simulink model "Design_5new_4weeks_01_06_MQTT"  (R2026a)
settings: Solver=FixedStepAuto  StopTime=2419200  FixedStep=300
undefined symbols (not defined in the file): m, n
libraries: mqttlib x7
(part 2 of 2)

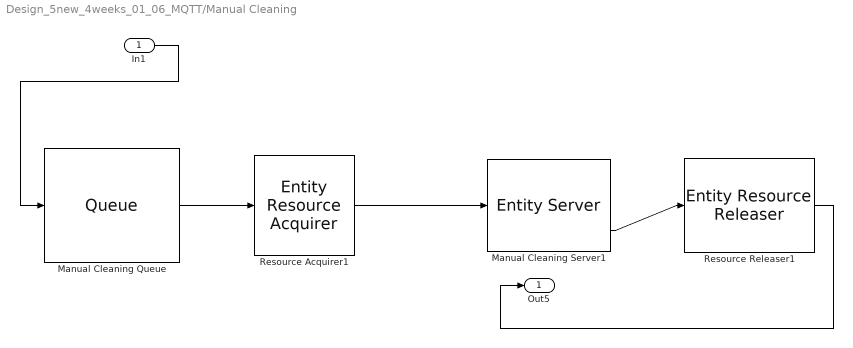
== system Design_5new_4weeks_01_06_MQTT/Manual Cleaning ==
  In1 : Inport
  Manual Cleaning Queue : Queue  InputPortMessageModes=m  OutputPortMessageModes=m
  Manual Cleaning Server1 : EntityServer  InputPortMessageModes=m  OutputPortMessageModes=n,m  Capacity=1  ServiceTimeValue=30*60  EntryAction=|  NumberEntitiesDeparted=on
      | %#codegen
      | 
      | % =========================================================
      | % MANUAL CLEANING PROCESS
      | % Supervisor Excel Values
      | % Simulink-safe version
      | % =========================================================
      | 
      | % Manual Cleaning completed
      | entity.prev_proc = 4;
      | 
      | % =========================================================
      | % FIX MANUAL BATCH ID
      | % =========================================================
      | % In the model, ManualBatchID sometimes becomes 0 here.
      | % If it is 0, use BatchID as the correct ManualBatchID.
      | % =========================================================
      | 
      | if entity.ManualBatchID == 0
      |     entity.ManualBatchID = entity.BatchID;
      | end
      | 
      | % =========================================================
      | % SUPERVISOR VALUES
      | % =========================================================
      | 
      | entity.operator_time_min = 30;              % min/batch
      | entity.capacity_L        = entity.part_volume;
      | entity.process_time_min  = 30;              % min
      | entity.power             = 0;               % kW
      | 
      | % =========================================================
      | % ENERGY CALCULATION
      | % =========================================================
      | 
      | entity.energy = 0;                          % kWh
      | 
      | % =========================================================
      | % ACCUMULATE TOTALS
      | % =========================================================
      | 
      | entity.total_energy = ...
      |     entity.total_energy + entity.energy;
      | 
      | entity.total_operator_min = ...
      |     entity.total_operator_min + entity.operator_time_min;
      | 
      | % =========================================================
      | % DEBUG PRINT
      | % =========================================================
      | 
      | fprintf(['[MANUAL CLEANING CHECK] ' ...
      |     'SourceID=%g | BuildID=%g | BatchID=%g | ' ...
      |     'ManualBatchID=%g | PartID=%g | ' ...
      |     'PrevProc=%g | Volume=%.2f | Capacity=%.2f | ' ...
      |     'ProcessTime=%.2f min | Operator=%.2f min | ' ...
      |     'Power=%.2f kW | Energy=%.3f kWh | ' ...
      |     'TotalEnergy=%.3f kWh | TotalOperator=%.3f min\n'], ...
      |     entity.SourceID, ...
      |     entity.BuildID, ...
      |     entity.BatchID, ...
      |     entity.ManualBatchID, ...
      |     entity.PartID, ...
      |     entity.prev_proc, ...
      |     entity.part_volume, ...
      |     entity.capacity_L, ...
      |     entity.process_time_min, ...
      |     entity.operator_time_min, ...
      |     entity.power, ...
      |     entity.energy, ...
      |     entity.total_energy, ...
      |     entity.total_operator_min);
      | 
      | % =========================================================
      | % MQTT PAYLOAD - MANUAL CLEANING
      | % FIWARE JSON object format
      | % =========================================================
      | 
      | payload = sprintf( ...
      |     '{"BuildID":%.0f,"BatchID":%.0f,"ManualBatchID":%.0f,"PartID":%.0f,"Volume":%.2f,"ProcessTime":%.2f,"Energy":%.3f}', ...
      |     entity.BuildID, ...
      |     entity.BatchID, ...
      |     entity.ManualBatchID, ...
      |     entity.PartID, ...
      |     entity.part_volume, ...
      |     entity.process_time_min, ...
      |     entity.energy);
      | 
      | payload = char(payload);
      | 
      | disp("[MANUAL CLEANING MQTT PAYLOAD]")
      | disp(payload)
      | 
      | % =========================================================
      | % CALL SIMULINK FUNCTION FOR MQTT PUBLISH
      | % This sends payload to MQTT Publish block
      | % =========================================================
      | 
      | publishManualCleaning( ...
      |     entity.BuildID, ...
      |     entity.BatchID, ...
      |     entity.ManualBatchID, ...
      |     entity.PartID, ...
      |     entity.part_volume, ...
      |     entity.process_time_min, ...
      |     entity.energy);
      settings: OutputPortMap=o0,o9
  Resource Acquirer1 : EntityResourceAcquirer  InputPortMessageModes=m  OutputPortMessageModes=m  ResourceName=operator_pool_1
      settings: OutputPortMap=o3
  Resource Releaser1 : EntityResourceReleaser  InputPortMessageModes=m  OutputPortMessageModes=m
  Out5 : Outport
  wires:
  Manual Cleaning Server1/2 -> Resource Releaser1/1
  In1/1 -> Manual Cleaning Queue/1
  Resource Acquirer1/1 -> Manual Cleaning Server1/1
  Manual Cleaning Queue/1 -> Resource Acquirer1/1
  Resource Releaser1/1 -> Out5/1

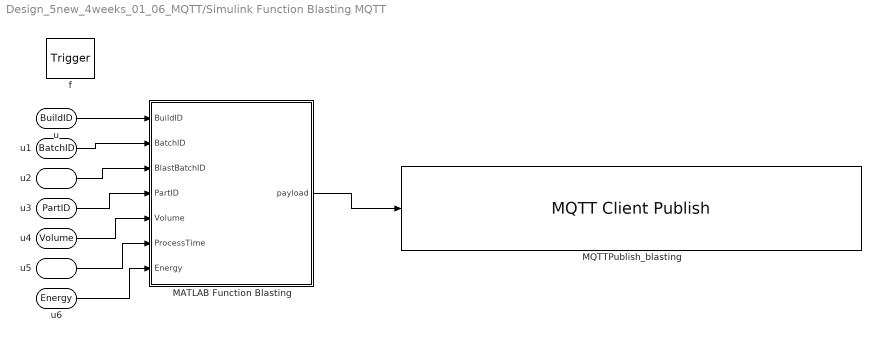
== system Design_5new_4weeks_01_06_MQTT/Simulink Function Blasting MQTT ==
  f : TriggerPort  TriggerType=function-call  IsSimulinkFunction=on  FunctionName=publishBlasting  VariantControl=(inherit)
  MATLAB Function Blasting : MATLAB Function  TreatAsAtomicUnit=on
  MQTTPublish_blasting : mqttlib/MQTT Client Publish  RetainClient=Fiware 1  ClientList=Fiware 1  TopicsTable={ '1', 'json/SLSProcess/BlastingMachine:001/attrs', '0', 'off' }  PublishOnDataChange=off  SampleTime=-1  TopicNames=json/SLSProcess/BlastingMachine:001/attrs  NumTopics=1  IsLib=0  BlkName=MQTT Client Publish
  u : ArgIn  DisableCoverage=on  ArgumentName=BuildID
  u1 : ArgIn  DisableCoverage=on  Port=2  ArgumentName=BatchID
  u2 : ArgIn  DisableCoverage=on  Port=3  ArgumentName=BlastBatchID
  u3 : ArgIn  DisableCoverage=on  Port=4  ArgumentName=PartID
  u4 : ArgIn  DisableCoverage=on  Port=5  ArgumentName=Volume
  u5 : ArgIn  DisableCoverage=on  Port=6  ArgumentName=ProcessTime
  u6 : ArgIn  DisableCoverage=on  Port=7  ArgumentName=Energy
  wires:
  u/1 -> MATLAB Function Blasting/1(BuildID)
  u1/1 -> MATLAB Function Blasting/2(BatchID)
  u2/1 -> MATLAB Function Blasting/3(BlastBatchID)
  u3/1 -> MATLAB Function Blasting/4(PartID)
  u4/1 -> MATLAB Function Blasting/5(Volume)
  u5/1 -> MATLAB Function Blasting/6(ProcessTime)
  u6/1 -> MATLAB Function Blasting/7(Energy)
  MATLAB Function Blasting/1(payload) -> MQTTPublish_blasting/1

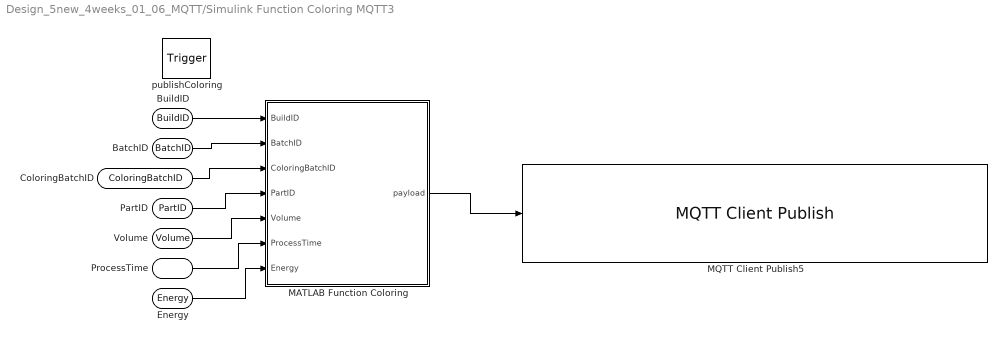
== system Design_5new_4weeks_01_06_MQTT/Simulink Function Coloring MQTT3 ==
  publishColoring : TriggerPort  TriggerType=function-call  IsSimulinkFunction=on  FunctionName=publishColoring  VariantControl=(inherit)
  MATLAB Function Coloring : MATLAB Function  TreatAsAtomicUnit=on
  MQTT Client Publish5 : mqttlib/MQTT Client Publish  RetainClient=Fiware 1  ClientList=Fiware 1  TopicsTable={ '1', 'json/SLSProcess/ColoringMachine:001/attrs', '0', 'off' }  PublishOnDataChange=off  SampleTime=-1  TopicNames=json/SLSProcess/ColoringMachine:001/attrs  NumTopics=1  IsLib=0  BlkName=MQTT Client Publish
  BuildID : ArgIn  DisableCoverage=on  ArgumentName=BuildID
  BatchID : ArgIn  DisableCoverage=on  Port=2  ArgumentName=BatchID
  ColoringBatchID : ArgIn  DisableCoverage=on  Port=3  ArgumentName=ColoringBatchID
  PartID : ArgIn  DisableCoverage=on  Port=4  ArgumentName=PartID
  Volume : ArgIn  DisableCoverage=on  Port=5  ArgumentName=Volume
  ProcessTime : ArgIn  DisableCoverage=on  Port=6  ArgumentName=ProcessTime
  Energy : ArgIn  DisableCoverage=on  Port=7  ArgumentName=Energy
  wires:
  BuildID/1 -> MATLAB Function Coloring/1(BuildID)
  BatchID/1 -> MATLAB Function Coloring/2(BatchID)
  ColoringBatchID/1 -> MATLAB Function Coloring/3(ColoringBatchID)
  PartID/1 -> MATLAB Function Coloring/4(PartID)
  Volume/1 -> MATLAB Function Coloring/5(Volume)
  ProcessTime/1 -> MATLAB Function Coloring/6(ProcessTime)
  Energy/1 -> MATLAB Function Coloring/7(Energy)
  MATLAB Function Coloring/1(payload) -> MQTT Client Publish5/1

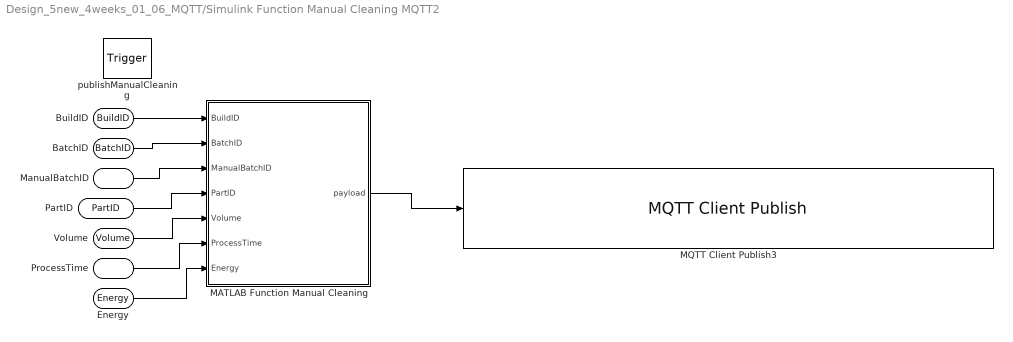
== system Design_5new_4weeks_01_06_MQTT/Simulink Function Manual Cleaning MQTT2 ==
  publishManualCleaning : TriggerPort  TriggerType=function-call  IsSimulinkFunction=on  FunctionName=publishManualCleaning  VariantControl=(inherit)
  MATLAB Function Manual Cleaning : MATLAB Function  TreatAsAtomicUnit=on
  MQTT Client Publish3 : mqttlib/MQTT Client Publish  RetainClient=Fiware 1  ClientList=Fiware 1  TopicsTable={ '1', 'json/SLSProcess/ManualCleaningMachine:001/attrs', '0', 'off' }  PublishOnDataChange=off  SampleTime=-1  TopicNames=json/SLSProcess/ManualCleaningMachine:001/attrs  NumTopics=1  IsLib=0  BlkName=MQTT Client Publish
  BuildID : ArgIn  DisableCoverage=on  ArgumentName=BuildID
  BatchID : ArgIn  DisableCoverage=on  Port=2  ArgumentName=BatchID
  ManualBatchID : ArgIn  DisableCoverage=on  Port=3  ArgumentName=ManualBatchID
  PartID : ArgIn  DisableCoverage=on  Port=4  ArgumentName=PartID
  Volume : ArgIn  DisableCoverage=on  Port=5  ArgumentName=Volume
  ProcessTime : ArgIn  DisableCoverage=on  Port=6  ArgumentName=ProcessTime
  Energy : ArgIn  DisableCoverage=on  Port=7  ArgumentName=Energy
  wires:
  BuildID/1 -> MATLAB Function Manual Cleaning/1(BuildID)
  BatchID/1 -> MATLAB Function Manual Cleaning/2(BatchID)
  ManualBatchID/1 -> MATLAB Function Manual Cleaning/3(ManualBatchID)
  PartID/1 -> MATLAB Function Manual Cleaning/4(PartID)
  Volume/1 -> MATLAB Function Manual Cleaning/5(Volume)
  ProcessTime/1 -> MATLAB Function Manual Cleaning/6(ProcessTime)
  Energy/1 -> MATLAB Function Manual Cleaning/7(Energy)
  MATLAB Function Manual Cleaning/1(payload) -> MQTT Client Publish3/1

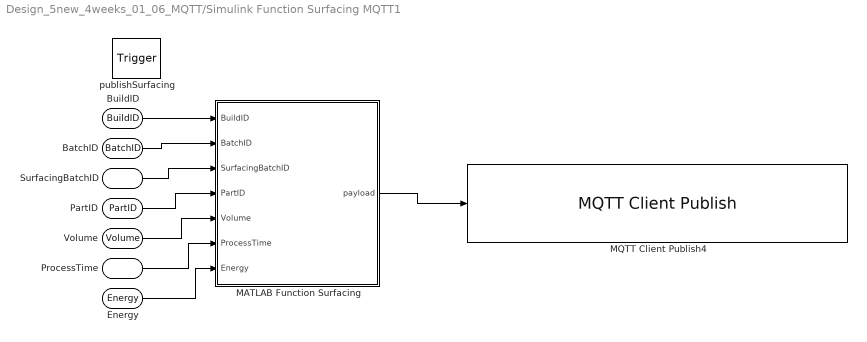
== system Design_5new_4weeks_01_06_MQTT/Simulink Function Surfacing MQTT1 ==
  publishSurfacing : TriggerPort  TriggerType=function-call  IsSimulinkFunction=on  FunctionName=publishSurfacing  VariantControl=(inherit)
  MATLAB Function Surfacing : MATLAB Function  TreatAsAtomicUnit=on
  MQTT Client Publish4 : mqttlib/MQTT Client Publish  RetainClient=Fiware 1  ClientList=Fiware 1  TopicsTable={ '1', 'json/SLSProcess/SurfacingMachine:001/attrs', '0', 'off' }  PublishOnDataChange=off  SampleTime=-1  TopicNames=json/SLSProcess/SurfacingMachine:001/attrs  NumTopics=1  IsLib=0  BlkName=MQTT Client Publish
  BuildID : ArgIn  DisableCoverage=on  ArgumentName=BuildID
  BatchID : ArgIn  DisableCoverage=on  Port=2  ArgumentName=BatchID
  SurfacingBatchID : ArgIn  DisableCoverage=on  Port=3  ArgumentName=SurfacingBatchID
  PartID : ArgIn  DisableCoverage=on  Port=4  ArgumentName=PartID
  Volume : ArgIn  DisableCoverage=on  Port=5  ArgumentName=Volume
  ProcessTime : ArgIn  DisableCoverage=on  Port=6  ArgumentName=ProcessTime
  Energy : ArgIn  DisableCoverage=on  Port=7  ArgumentName=Energy
  wires:
  BuildID/1 -> MATLAB Function Surfacing/1(BuildID)
  BatchID/1 -> MATLAB Function Surfacing/2(BatchID)
  SurfacingBatchID/1 -> MATLAB Function Surfacing/3(SurfacingBatchID)
  PartID/1 -> MATLAB Function Surfacing/4(PartID)
  Volume/1 -> MATLAB Function Surfacing/5(Volume)
  ProcessTime/1 -> MATLAB Function Surfacing/6(ProcessTime)
  Energy/1 -> MATLAB Function Surfacing/7(Energy)
  MATLAB Function Surfacing/1(payload) -> MQTT Client Publish4/1

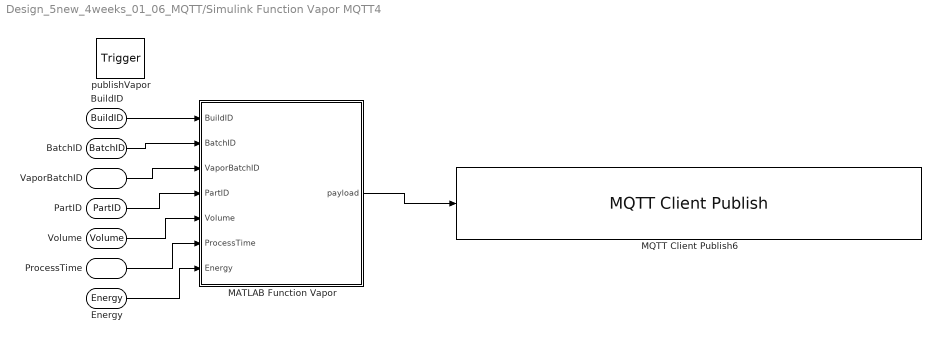
== system Design_5new_4weeks_01_06_MQTT/Simulink Function Vapor MQTT4 ==
  publishVapor : TriggerPort  TriggerType=function-call  IsSimulinkFunction=on  FunctionName=publishVapor  VariantControl=(inherit)
  MATLAB Function Vapor : MATLAB Function  TreatAsAtomicUnit=on
  MQTT Client Publish6 : mqttlib/MQTT Client Publish  RetainClient=Fiware 1  ClientList=Fiware 1  TopicsTable={ '1', 'json/SLSProcess/VaporSmoothingMachine:001/attrs', '0', 'off' }  PublishOnDataChange=off  SampleTime=-1  TopicNames=json/SLSProcess/VaporSmoothingMachine:001/attrs  NumTopics=1  IsLib=0  BlkName=MQTT Client Publish
  BuildID : ArgIn  DisableCoverage=on  ArgumentName=BuildID
  BatchID : ArgIn  DisableCoverage=on  Port=2  ArgumentName=BatchID
  VaporBatchID : ArgIn  DisableCoverage=on  Port=3  ArgumentName=VaporBatchID
  PartID : ArgIn  DisableCoverage=on  Port=4  ArgumentName=PartID
  Volume : ArgIn  DisableCoverage=on  Port=5  ArgumentName=Volume
  ProcessTime : ArgIn  DisableCoverage=on  Port=6  ArgumentName=ProcessTime
  Energy : ArgIn  DisableCoverage=on  Port=7  ArgumentName=Energy
  wires:
  BuildID/1 -> MATLAB Function Vapor/1(BuildID)
  BatchID/1 -> MATLAB Function Vapor/2(BatchID)
  VaporBatchID/1 -> MATLAB Function Vapor/3(VaporBatchID)
  PartID/1 -> MATLAB Function Vapor/4(PartID)
  Volume/1 -> MATLAB Function Vapor/5(Volume)
  ProcessTime/1 -> MATLAB Function Vapor/6(ProcessTime)
  Energy/1 -> MATLAB Function Vapor/7(Energy)
  MATLAB Function Vapor/1(payload) -> MQTT Client Publish6/1

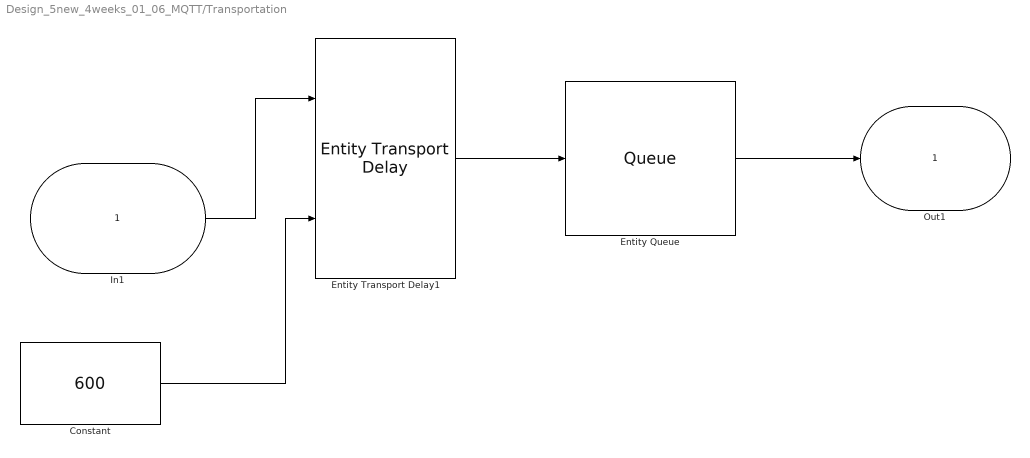
== system Design_5new_4weeks_01_06_MQTT/Transportation ==
  In1 : Inport
  Constant : Constant  Value=600
  Entity Transport Delay1 : EntityTransportDelay  InputPortMessageModes=m,n  OutputPortMessageModes=m
  Entity Queue : Queue  InputPortMessageModes=m  OutputPortMessageModes=m
  Out1 : Outport
  wires:
  Entity Transport Delay1/1 -> Entity Queue/1
  In1/1 -> Entity Transport Delay1/1
  Constant/1 -> Entity Transport Delay1/2
  Entity Queue/1 -> Out1/1

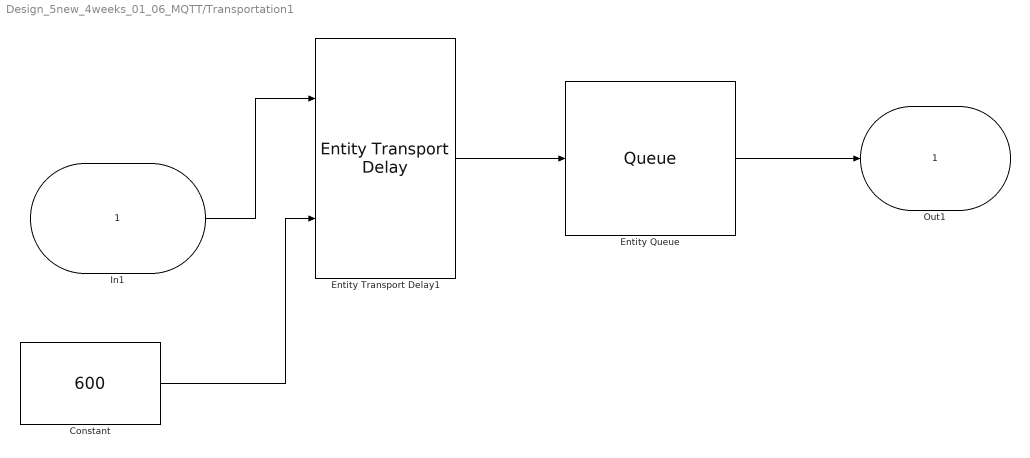
== system Design_5new_4weeks_01_06_MQTT/Transportation1 ==
  In1 : Inport
  Constant : Constant  Value=600
  Entity Transport Delay1 : EntityTransportDelay  InputPortMessageModes=m,n  OutputPortMessageModes=m
  Entity Queue : Queue  InputPortMessageModes=m  OutputPortMessageModes=m
  Out1 : Outport
  wires:
  Entity Transport Delay1/1 -> Entity Queue/1
  In1/1 -> Entity Transport Delay1/1
  Constant/1 -> Entity Transport Delay1/2
  Entity Queue/1 -> Out1/1

== matlab function Design_5new_4weeks_01_06_MQTT/Simulink Function Manual Cleaning MQTT2/MATLAB Function Manual Cleaning ==
  data: payload output string; BuildID input; BatchID input; ManualBatchID input; PartID input; Volume input; ProcessTime input; Energy input

function payload = fcn(BuildID,BatchID,ManualBatchID,PartID,Volume,ProcessTime,Energy)
%#codegen

disp("[MANUAL CLEANING MQTT FUNCTION CALLED]")

% If ManualBatchID becomes 0, use BatchID instead
if ManualBatchID == 0
    ManualBatchID = BatchID;
end

payload = string(sprintf( ...
    '{"BuildID":%.0f,"BatchID":%.0f,"ManualBatchID":%.0f,"PartID":%.0f,"Volume":%.2f,"ProcessTime":%.2f,"Energy":%.3f}', ...
    BuildID, BatchID, ManualBatchID, PartID, Volume, ProcessTime, Energy));

disp(payload)

end

== matlab function Design_5new_4weeks_01_06_MQTT/Simulink Function Vapor MQTT4/MATLAB Function Vapor ==
  data: payload output string; BuildID input; BatchID input; VaporBatchID input; PartID input; Volume input; ProcessTime input; Energy input
function payload = fcn(BuildID,BatchID,VaporBatchID,PartID,Volume,ProcessTime,Energy)
%#codegen

payload = string(sprintf( ...
    '{"BuildID":%.0f,"BatchID":%.0f,"VaporBatchID":%.0f,"PartID":%.0f,"Volume":%.2f,"ProcessTime":%.2f,"Energy":%.3f}', ...
    BuildID, BatchID, VaporBatchID, PartID, Volume, ProcessTime, Energy));

disp("[VAPOR PAYLOAD CREATED]")
disp(payload)

end

== matlab function Design_5new_4weeks_01_06_MQTT/Simulink Function Surfacing MQTT1/MATLAB Function Surfacing ==
  data: payload output string; BuildID input; BatchID input; SurfacingBatchID input; PartID input; Volume input; ProcessTime input; Energy input

function payload = fcn(BuildID,BatchID,SurfacingBatchID,PartID,Volume,ProcessTime,Energy)
%#codegen

payload = string(sprintf( ...
    '{"BuildID":%.0f,"BatchID":%.0f,"SurfacingBatchID":%.0f,"PartID":%.0f,"Volume":%.2f,"ProcessTime":%.2f,"Energy":%.3f}', ...
    BuildID, BatchID, SurfacingBatchID, PartID, Volume, ProcessTime, Energy));

disp("[SURFACING PAYLOAD CREATED]")
disp(payload)

end

== matlab function Design_5new_4weeks_01_06_MQTT/MATLAB Function 3 ==
  data: t input; dt output



function dt = fcn_printer2(t)
%#codegen

SEC_PER_DAY = 24*3600;
rel_sec = 8*3600;    % Same as Printer 1 → 08:00 AM
epsT = 1e-9;

day  = floor(t/SEC_PER_DAY);
tod  = mod(t, SEC_PER_DAY);

next_day = day;

while true
    ndow  = mod(next_day,7);      % day of week
    nweek = floor(next_day/7);    % week index

    % Skip weekends
    if ndow == 5 || ndow == 6
        next_day = next_day + 1;
        continue;
    end

    % Skip first Monday of week 1
    if (nweek == 0) && (ndow == 0)
        next_day = next_day + 1;
        continue;
    end

    % Check today's time
    if next_day == day
        if tod < rel_sec - epsT
            break;   % release today at 08:00
        else
            next_day = next_day + 1;
            continue;
        end
    else
        break;
    end
end

next_release = next_day*SEC_PER_DAY + rel_sec;

% Ensure positive time step
dt = max(next_release - t, 1e-6);

end

== matlab function Design_5new_4weeks_01_06_MQTT/MATLAB Function 4 ==
  data: t input; cap output




function cap = operator_capacity_p2(t)
%#codegen

SEC_PER_DAY = 24*3600;

day = floor(t/SEC_PER_DAY);     % Day index
tod = mod(t, SEC_PER_DAY);      % Time of day (seconds)
dow = mod(day,7);               % Day of week (0=Mon,...,6=Sun)
week = floor(day/7);            % Week index

% --- Weekend: no operator ---
if dow >= 5
    cap = 0;
    return;
end

% --- Special case: First Monday (week 0) ---
if (week == 0) && (dow == 0)
    % Only 12:00–16:00
    if tod >= 12*3600 && tod < 16*3600
        cap = 1;
    else
        cap = 0;
    end
else
    % Normal weekdays: 08:00–16:00
    if tod >= 8*3600 && tod < 16*3600
        cap = 1;
    else
        cap = 0;
    end
end

end

== matlab function Design_5new_4weeks_01_06_MQTT/MATLAB Function 1 ==
  data: t input; dt output



function dt = fcn(t)
%#codegen

SEC_PER_DAY = 24*3600;
rel_sec = 8*3600;      % 08:00
epsT = 1e-9;

day  = floor(t/SEC_PER_DAY);
tod  = mod(t, SEC_PER_DAY);

next_day = day;

while true
    ndow  = mod(next_day,7);
    nweek = floor(next_day/7);

    if ndow == 5 || ndow == 6
        next_day = next_day + 1;
        continue;
    end

    if (nweek == 0) && (ndow == 0)
        next_day = next_day + 1;
        continue;
    end

    if next_day == day
        if tod < rel_sec - epsT
            break;
        else
            next_day = next_day + 1;
            continue;
        end
    else
        break;
    end
end

next_release = next_day*SEC_PER_DAY + rel_sec;
dt = max(next_release - t, 1e-6);

end

== matlab function Design_5new_4weeks_01_06_MQTT/MATLAB Function 2 ==
  data: t input; cap output




function cap = operator_capacity_p1(t)
%#codegen

SEC_PER_DAY = 24*3600;

day = floor(t/SEC_PER_DAY);     % Day index
tod = mod(t, SEC_PER_DAY);      % Time of day (seconds)
dow = mod(day,7);               % Day of week (0=Mon,...,6=Sun)
week = floor(day/7);            % Week index

% --- Weekend: no operator ---
if dow >= 5
    cap = 0;
    return;
end

% --- Special case: First Monday (week 0) ---
if (week == 0) && (dow == 0)
    % Only 12:00–16:00
    if tod >= 12*3600 && tod < 16*3600
        cap = 1;
    else
        cap = 0;
    end
else
    % Normal weekdays: 08:00–16:00
    if tod >= 8*3600 && tod < 16*3600
        cap = 1;
    else
        cap = 0;
    end
end

end

== matlab function Design_5new_4weeks_01_06_MQTT/Simulink Function Coloring MQTT3/MATLAB Function Coloring ==
  data: payload output string; BuildID input; BatchID input; ColoringBatchID input; PartID input; Volume input; ProcessTime input; Energy input

function payload = fcn(BuildID,BatchID,ColoringBatchID,PartID,Volume,ProcessTime,Energy)
%#codegen

payload = string(sprintf( ...
    '{"BuildID":%.0f,"BatchID":%.0f,"ColoringBatchID":%.0f,"PartID":%.0f,"Volume":%.2f,"ProcessTime":%.2f,"Energy":%.3f}', ...
    BuildID, BatchID, ColoringBatchID, PartID, Volume, ProcessTime, Energy));

disp("[COLORING PAYLOAD CREATED]")
disp(payload)

end

== matlab function Design_5new_4weeks_01_06_MQTT/Simulink Function Blasting MQTT/MATLAB Function Blasting ==
  data: payload output string; BuildID input; BatchID input; BlastBatchID input; PartID input; Volume input; ProcessTime input; Energy input

function payload = fcn(BuildID,BatchID,BlastBatchID,PartID,Volume,ProcessTime,Energy)
%#codegen

disp("[BLASTING MQTT FUNCTION CALLED]")

payload = string(sprintf( ...
    '{"BuildID":%.0f,"BatchID":%.0f,"BlastBatchID":%.0f,"PartID":%.0f,"Volume":%.2f,"ProcessTime":%.2f,"Energy":%.3f}', ...
    BuildID, BatchID, BlastBatchID, PartID, Volume, ProcessTime, Energy));

disp(payload)

end
